simulink model "Simlink"  (R2018b)
settings: Solver=ode3  StartTime=0.0  StopTime=10.0  FixedStep=0.01  RelTol=1e-3
undefined symbols (not defined in the file): DiscIntNeverNeededParam
settings Model: Creator=a4lfr  LastModifiedBy=a4lfr

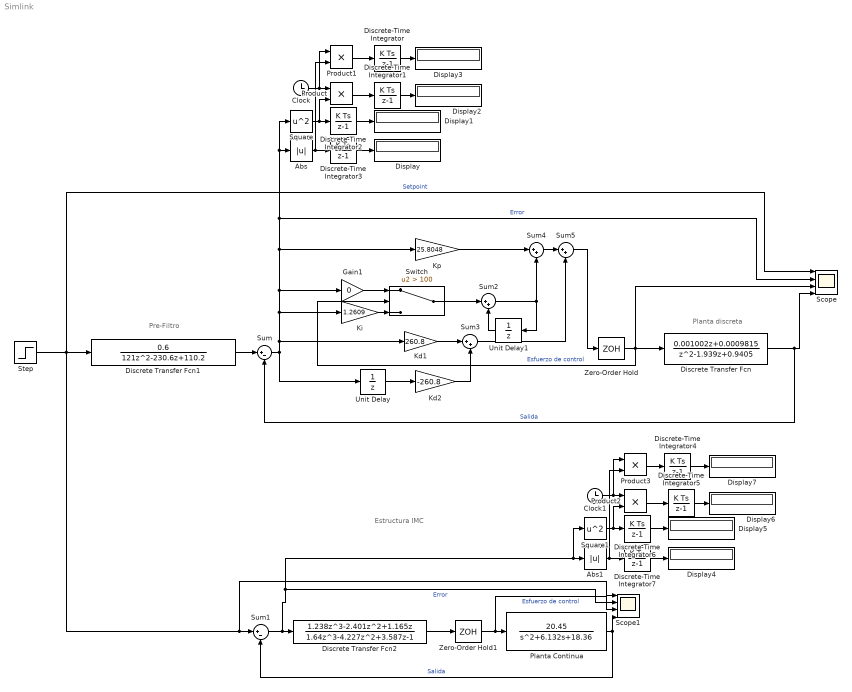
== system Simlink ==
  note: Planta discreta
  note: Pre-Filtro
  note: Estructura IMC
  Abs : Abs
  Abs1 : Abs
  Clock : Clock
  Clock1 : Clock
  Discrete Transfer Fcn : DiscreteTransferFcn  Numerator=[0.001002,0.0009815]  Denominator=[1,-1.939,0.9405]
  Discrete Transfer Fcn1 : DiscreteTransferFcn  Numerator=[0,0,0.6]  Denominator=[121,-230.6,110.2]
  Discrete Transfer Fcn2 : DiscreteTransferFcn  Numerator=[1.238,-2.401,1.165,0]  Denominator=[1.64,-4.227,3.587,-1]
  Discrete-Time Integrator{,1..7} (8 alike) : DiscreteIntegrator  SampleTime=-1  ICPrevOutput=DiscIntNeverNeededParam  ICPrevScaledInput=DiscIntNeverNeededParam
  Display{,1..7} (8 alike) : Display
  Gain1 : Gain  Gain=0
  "Kd1 " : Gain  Gain=260.8
  Kd2 : Gain  Gain=-260.8
  Ki : Gain  Gain=1.2609
  Kp : Gain  Gain=25.8048
  Planta Continua : TransferFcn  Numerator=[0,0,20.45]  Denominator=[1,6.132,18.36]
  Product{,1..3} (4 alike) : Product
  Scope : Scope  NumInputPorts=4
  Scope1 : Scope  NumInputPorts=4
  Square : Math  Operator=square  SaturateOnIntegerOverflow=on
  Square1 : Math  Operator=square  SaturateOnIntegerOverflow=on
  Step : Step  SampleTime=0
  Sum : Sum  Inputs=|+-
  Sum1 : Sum  Inputs=|+-
  Sum{2..5} (4 alike) : Sum  Inputs=|++
  Switch : Switch  Criteria=u2 > Threshold  Threshold=100
  Unit Delay : UnitDelay  SampleTime=-1
  Unit Delay1 : UnitDelay  SampleTime=-1
  Zero-Order Hold : ZeroOrderHold  SampleTime=0.01
  Zero-Order Hold1 : ZeroOrderHold  SampleTime=0.01
  wires:
  Sum/1 -> Ki/1, Square/1, Abs/1, Scope/2, Kp/1, Gain1/1, "Kd1 "/1, Unit Delay/1  "Error"
  Zero-Order Hold/1 -> Switch/2, Discrete Transfer Fcn/1, Scope/3  "Esfuerzo de control"
  Discrete Transfer Fcn1/1 -> Sum/1
  Step/1 -> Scope1/1, Sum1/1, Scope/1, Discrete Transfer Fcn1/1  "Setpoint"
  Planta Continua/1 -> Sum1/2, Scope1/4  "Salida"
  Zero-Order Hold1/1 -> Scope1/3, Planta Continua/1  "Esfuerzo de control"
  Discrete Transfer Fcn2/1 -> Zero-Order Hold1/1
  Abs/1 -> Discrete-Time Integrator3/1, Product1/2
  Square/1 -> Discrete-Time Integrator2/1, Product/2
  Clock/1 -> Product1/1, Product/1
  Product/1 -> Discrete-Time Integrator1/1
  Product1/1 -> Discrete-Time Integrator/1
  Discrete-Time Integrator/1 -> Display3/1
  Discrete-Time Integrator4/1 -> Display7/1
  Product3/1 -> Discrete-Time Integrator4/1
  Product2/1 -> Discrete-Time Integrator5/1
  Clock1/1 -> Product2/1, Product3/1
  Discrete-Time Integrator6/1 -> Display5/1
  Square1/1 -> Discrete-Time Integrator6/1, Product2/2
  Abs1/1 -> Discrete-Time Integrator7/1, Product3/2
  Sum1/1 -> Abs1/1, Square1/1, Scope1/2, Discrete Transfer Fcn2/1  "Error"
  Discrete-Time Integrator1/1 -> Display2/1
  Discrete-Time Integrator2/1 -> Display1/1
  Discrete-Time Integrator3/1 -> Display/1
  Discrete-Time Integrator5/1 -> Display6/1
  Discrete-Time Integrator7/1 -> Display4/1
  Discrete Transfer Fcn/1 -> Sum/2, Scope/4  "Salida"
  Unit Delay/1 -> Kd2/1
  Sum2/1 -> Sum4/2, Unit Delay1/1
  Unit Delay1/1 -> Sum2/2
  "Kd1 "/1 -> Sum3/1
  Kd2/1 -> Sum3/2
  Kp/1 -> Sum4/1
  Sum4/1 -> Sum5/1
  Sum3/1 -> Sum5/2
  Sum5/1 -> Zero-Order Hold/1
  Gain1/1 -> Switch/1
  Switch/1 -> Sum2/1
  Ki/1 -> Switch/3
